simulink model "Pendulum_and_frictions_75"  (Simulink 7.0)
settings: Solver=FixedStepDiscrete  SolverMode=SingleTasking  StartTime=0.0  StopTime=50  FixedStep=Ts  RelTol=1e-3
values from neighbouring files (symbols this model uses):
  Cm = Cmm    [MMCE.m]
  F = zeros(n)    [MMCE.m]    (also in yalmip_lmi_reg.m = F + set(kron(Lreg,Y) + kron(Mreg,(A*Y-B*W)') + kron(Mreg',(A)
  G = zeros(n,q)    [MMCE.m]
  H = zeros(n)    [MMCE.m]
  J = zeros(n,p)    [MMCE.m]
  K = zeros(n,q)    [MMCE.m]
  L = Rounding_Matrix(real(L_Bec_Ost))    [Becker_Ostertag.m]    (also in Falb_Wolovich_or_Roppenecker.m = Rounding_Matrix(L_decoupling); MMCE.m = input('Matrix L = '); Roppenecker.m = Rounding_Matrix(real(L_Roppenecker)))
  M = [A-lambdades(i)*eye(n) -B]    [Choice_Eigenvec_Paramvec.m]    (also in Falb_Wolovich_or_Roppenecker.m = inv(Dstar)*diag([knum]); MMCE.m = inv(G_CL),)
  n = size(A,1)    [Becker_Ostertag.m]    (also in Falb_Wolovich_or_Roppenecker.m; MMCE.m; Responses.m = size(A_CL,1); Roppenecker.m)
  p = size(B,2)    [Becker_Ostertag.m]    (also in Falb_Wolovich_or_Roppenecker.m; MMCE.m = size(Bc,2); Responses.m; Roppenecker.m)
  Ts = 1    [MMCE.m]
  x0 = xx0    [MMCE.m]    (also in Responses.m = as above) (Y/N)? [N] --> ','s'); yalmip_lmi_reg.m = input('  Enter a real number:  '))
undefined symbols (not defined in the file or in its folder): Gamma, Phi
libraries: simulink x5
settings Model: Creator=Eric  LastModifiedBy=Eric  ExtModeTrigDuration=10000  ExtModeArchiveMode=auto  ExtModeArchiveFileName=SSControl_threshold_then_obs  ExtModeArchiveDirName=E:\MATLABR11\Perso\Logs  ExtModeAutoIncOneShot=on
settings DataIOCC: LimitDataPoints=off  SignalLoggingName=sigsOut
settings OptimizationCC: BooleanDataType=off
settings DebuggingCC: SaveWithParameterizedLinksMsg=none  SignalResolutionControl=TryResolveAllWithWarning  SolverPrmCheckMsg=none  MultiTaskDSMMsg=warning  MultiTaskCondExecSysMsg=none  StrictBusMsg=None
settings HardwareCC: TargetUnknown=on
settings RTWCC: SystemTargetFile=rtwin.tlc  TemplateMakefile=rtwintmf  ProcessScript=rtwin_make_rtw_hook  IncludeERTFirstTime=on
settings RTWinTargetCC: TargetFcnLib=ansi_tfl_tmw.mat  GenFloatMathFcnCalls=ANSI_C  ModelReferenceCompliant=off  CompOptLevelCompliant=off  PortableWordSizes=off  CCOptimize=on

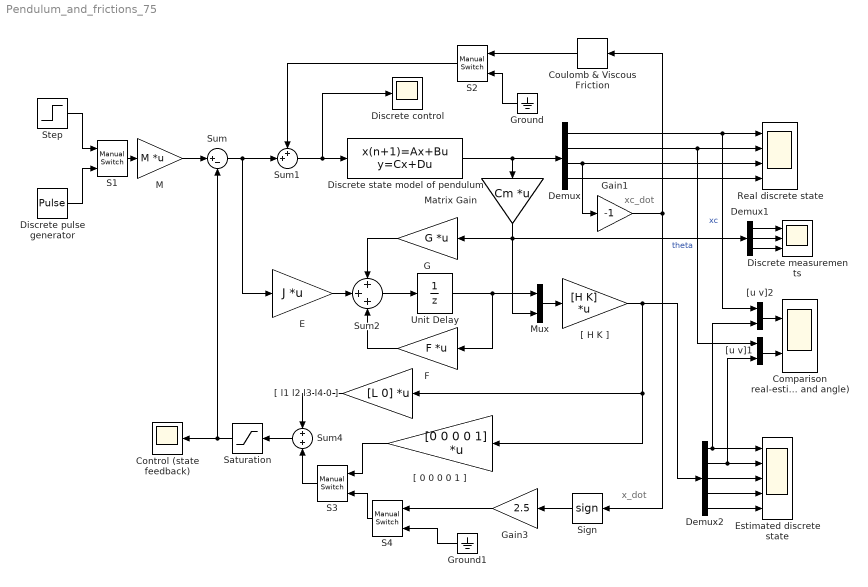
== system Pendulum_and_frictions_75 ==
  note: xc_dot
  note: x_dot
  Comparison real-estimate (position and angle) : Scope  NumInputPorts=2
      settings: YMin=-0.1~-0.2  YMax=0.3~0.2  SaveName=CompareScope  MaxDataPoints=10000
  Control (state feedback) : Scope
      settings: YMin=-10  YMax=10  MaxDataPoints=10000
  Coulomb & Viscous Friction : simulink/Discontinuities/Coulomb & Viscous Friction  Orientation=left  SystemSampleTime=-1  offset=2.5  gain=0
  Demux : Demux  Outputs=n
  Demux1 : Demux  Outputs=q
  Demux2 : Demux  Outputs=5
  Discrete measurements : Scope  NumInputPorts=3
      settings: YMin=-10~-5~-5  YMax=10~5~5  SaveName=MeasurementScope  MaxDataPoints=10000
  Discrete pulse generator : DiscretePulseGenerator  Amplitude=2  Period=1000  PulseWidth=500  SampleTime=Ts
  Discrete control : Scope
      settings: YMin=-2.5  YMax=3  SaveName=ControlScope  MaxDataPoints=10000
  Discrete state model of pendulum : DiscreteStateSpace  A=Phi  B=Gamma  C=eye(n)  D=zeros(n,p)  X0=x0  SampleTime=Ts
  E : Gain  Gain=J  Multiplication=Matrix(K*u)  ParameterDataType=sfix(16)  ParameterScaling=2^0  OutDataType=sfix(16)  OutScaling=2^0  SaturateOnIntegerOverflow=on
  Estimated discrete state : Scope  NumInputPorts=5
      settings: YMin=-10~-5~-5~-5~-5  YMax=10~5~5~5~5  SaveName=EstimateScope  MaxDataPoints=10000
  F : Gain  Orientation=left  Gain=F  Multiplication=Matrix(K*u)  ParameterDataType=sfix(16)  ParameterScaling=2^0  OutDataType=sfix(16)  OutScaling=2^0  SaturateOnIntegerOverflow=on
  G : Gain  Orientation=left  Gain=G  Multiplication=Matrix(K*u)  ParameterDataType=sfix(16)  ParameterScaling=2^0  OutDataType=sfix(16)  OutScaling=2^0  SaturateOnIntegerOverflow=on
  Gain1 : Gain  Gain=-1  ParameterDataType=sfix(16)  ParameterScaling=2^0  OutDataType=sfix(16)  OutScaling=2^0  SaturateOnIntegerOverflow=on
  Gain3 : Gain  Orientation=left  Gain=2.5  ParameterDataType=sfix(16)  ParameterScaling=2^0  OutDataType=sfix(16)  OutScaling=2^0  SaturateOnIntegerOverflow=on
  Ground : Ground  Orientation=left
  Ground1 : Ground  Orientation=left
  M : Gain  Gain=M  Multiplication=Matrix(K*u)  ParameterDataType=sfix(16)  ParameterScaling=2^0  OutDataType=sfix(16)  OutScaling=2^0  SaturateOnIntegerOverflow=on
  Matrix Gain : Gain  Orientation=down  Gain=Cm  Multiplication=Matrix(K*u)  ParameterDataType=sfix(16)  ParameterScaling=2^0  OutDataType=sfix(16)  OutScaling=2^0  SaturateOnIntegerOverflow=on
  Mux : Mux  Inputs=2
  Real discrete state : Scope  NumInputPorts=4
      settings: YMin=-3~-5~-5~-5  YMax=5~4~5~5  SaveName=StateScope  MaxDataPoints=10000
  S1 : simulink/Signal Routing/Manual Switch  SystemSampleTime=-1  sw=0  action=0  varsize=off
  S2 : simulink/Signal Routing/Manual Switch  Orientation=left  SystemSampleTime=-1  sw=1  action=0  varsize=off
  S3 : simulink/Signal Routing/Manual Switch  Orientation=left  SystemSampleTime=-1  sw=0  action=0  varsize=off
  S4 : simulink/Signal Routing/Manual Switch  Orientation=left  SystemSampleTime=-1  sw=0  action=0  varsize=off
  Saturation : Saturate  Orientation=left  UpperLimit=9.9  LowerLimit=-9.9
  Sign : Signum  Orientation=left
  Step : Step  Time=100*Ts  SampleTime=Ts
  Sum : Sum  Inputs=|+-  OutDataType=sfix(16)  OutScaling=2^0  SaturateOnIntegerOverflow=on  InputSameDT=on
  Sum1 : Sum  Inputs=++|  OutDataType=sfix(16)  OutScaling=2^0  SaturateOnIntegerOverflow=on  InputSameDT=on
  Sum2 : Sum  Inputs=+++  OutDataType=sfix(16)  OutScaling=2^0  SaturateOnIntegerOverflow=on  InputSameDT=on
  Sum4 : Sum  Orientation=left  OutDataType=sfix(16)  OutScaling=2^0  SaturateOnIntegerOverflow=on  InputSameDT=on
  Unit Delay : UnitDelay  SampleTime=Ts
  "[ 0 0 0 0 1 ]" : Gain  Orientation=left  Gain=[0 0 0 0 1]  Multiplication=Matrix(K*u)  ParameterDataType=sfix(16)  ParameterScaling=2^0  OutDataType=sfix(16)  OutScaling=2^0  SaturateOnIntegerOverflow=on
  "[ H K ]" : Gain  Gain=[H K]  Multiplication=Matrix(K*u)  ParameterDataType=sfix(16)  ParameterScaling=2^0  OutDataType=sfix(16)  OutScaling=2^0  SaturateOnIntegerOverflow=on
  "[ l1 l2 l3 l4 0 ]" : Gain  Orientation=left  Gain=[L 0]  Multiplication=Matrix(K*u)  ParameterDataType=sfix(16)  ParameterScaling=2^0  OutDataType=sfix(16)  OutScaling=2^0  SaturateOnIntegerOverflow=on
  "[u v]1" : Mux  Inputs=2
  "[u v]2" : Mux  Inputs=2
  wires:
  Demux/2 -> Real discrete state/2, "[u v]1"/1  "theta"
  Demux/3 -> Gain1/1, Real discrete state/3
  S1/1 -> M/1
  Step/1 -> S1/1
  Discrete pulse generator/1 -> S1/2
  Coulomb & Viscous Friction/1 -> S2/1
  Ground/1 -> S2/2
  S2/1 -> Sum1/1
  Sum1/1 -> Discrete control/1, Discrete state model of pendulum/1
  Sum2/1 -> Unit Delay/1
  Unit Delay/1 -> F/1, Mux/1
  Mux/1 -> "[ H K ]"/1
  F/1 -> Sum2/3
  E/1 -> Sum2/2
  G/1 -> Sum2/1
  Sign/1 -> Gain3/1
  Gain3/1 -> S4/1
  Sum4/1 -> Saturation/1
  S3/1 -> Sum4/2
  Saturation/1 -> Control (state feedback)/1, Sum/2
  "[ 0 0 0 0 1 ]"/1 -> S3/1
  "[ H K ]"/1 -> "[ 0 0 0 0 1 ]"/1, "[ l1 l2 l3 l4 0 ]"/1, Demux2/1
  "[ l1 l2 l3 l4 0 ]"/1 -> Sum4/1
  M/1 -> Sum/1
  Sum/1 -> Sum1/2, E/1
  Ground1/1 -> S4/2
  S4/1 -> S3/2
  Discrete state model of pendulum/1 -> Demux/1, Matrix Gain/1
  Matrix Gain/1 -> G/1, Mux/2, Demux1/1
  Demux/1 -> Real discrete state/1, "[u v]2"/1  "xc"
  Gain1/1 -> Sign/1, Coulomb & Viscous Friction/1
  Demux1/1 -> Discrete measurements/1
  Demux1/2 -> Discrete measurements/2
  Demux2/1 -> Estimated discrete state/1, "[u v]2"/2
  Demux2/2 -> Estimated discrete state/2, "[u v]1"/2
  Demux2/3 -> Estimated discrete state/3
  Demux2/4 -> Estimated discrete state/4
  Demux2/5 -> Estimated discrete state/5
  Demux/4 -> Real discrete state/4
  "[u v]2"/1 -> Comparison real-estimate (position and angle)/1
  "[u v]1"/1 -> Comparison real-estimate (position and angle)/2
  Demux1/3 -> Discrete measurements/3
